simulink library "NMHA_lib"  (Simulink 7.5)
settings: Solver=ode45  StartTime=0.0  StopTime=10.0  RelTol=1e-3
values from neighbouring files (symbols this model uses):
  pNMHA_cnt_CANSleepDely_C = Simulink.Parameter    [NMHA_par.m]
  pNMHA_cnt_VCUSleepDely_C = Simulink.Parameter    [NMHA_par.m]
undefined symbols (not defined in the file or in its folder): p_bool_False_M, p_bool_True_M, VMMCoorrStsTyp
libraries: BaseOperationLib_Browser x6, simulink x1
settings Model: Creator=wuaibin  LastModifiedBy=wuaibin

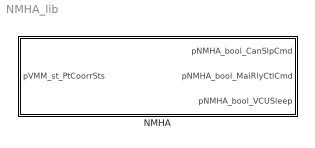
== system NMHA_lib ==
  NMHA : Subsystem  TreatAsAtomicUnit=on

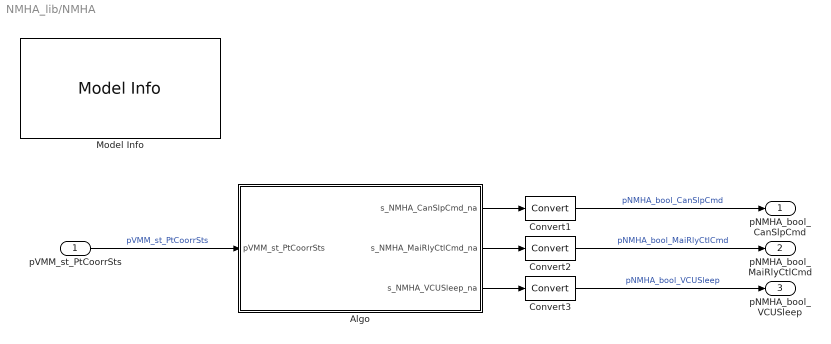
== system NMHA_lib/NMHA ==
  pVMM_st_PtCoorrSts : Inport  OutDataType=fixdt(1, 16)  OutScaling=2^0
  Algo : Subsystem
  Convert1 : DataTypeConversion  OutDataType=fixdt(1, 16)  OutScaling=2^0
  Convert2 : DataTypeConversion  OutDataType=fixdt(1, 16)  OutScaling=2^0
  Convert3 : DataTypeConversion  OutDataType=fixdt(1, 16)  OutScaling=2^0
  Model Info : simulink/Model-Wide Utilities/Model Info  SystemSampleTime=-1  InitialBlockCM=None  BlockCM=None  Frame=on  DisplayStringWithTags=Model Info\nCreated: %<Created>\nCreator: wuaibin  HorizontalTextAlignment=Center  LeftAlignmentValue=0.5  SourceBlockDiagram=HQEV_HCU  TagMaxNumber=20
  pNMHA_bool_CanSlpCmd : Outport  OutDataType=fixdt(1, 16)  OutScaling=2^0
  pNMHA_bool_MaiRlyCtlCmd : Outport  Port=2  OutDataType=fixdt(1, 16)  OutScaling=2^0
  pNMHA_bool_VCUSleep : Outport  Port=3  OutDataType=fixdt(1, 16)  OutScaling=2^0
  wires:
  pVMM_st_PtCoorrSts/1 -> Algo/1(pVMM_st_PtCoorrSts)  "pVMM_st_PtCoorrSts"
  Algo/1(s_NMHA_CanSlpCmd_na) -> Convert1/1
  Convert1/1 -> pNMHA_bool_CanSlpCmd/1  "pNMHA_bool_CanSlpCmd"
  Algo/2(s_NMHA_MaiRlyCtlCmd_na) -> Convert2/1
  Convert2/1 -> pNMHA_bool_MaiRlyCtlCmd/1  "pNMHA_bool_MaiRlyCtlCmd"
  Algo/3(s_NMHA_VCUSleep_na) -> Convert3/1
  Convert3/1 -> pNMHA_bool_VCUSleep/1  "pNMHA_bool_VCUSleep"

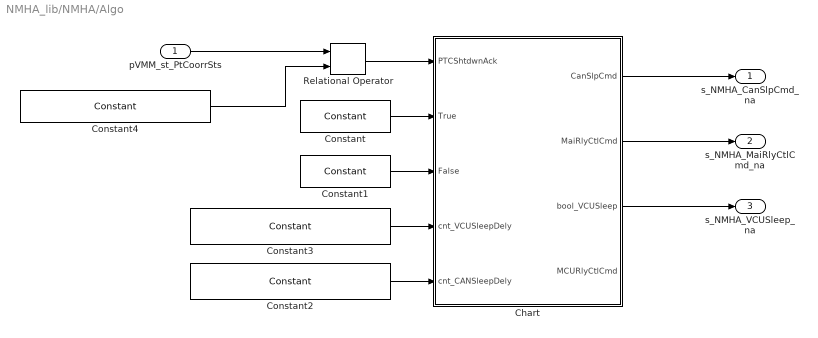
== system NMHA_lib/NMHA/Algo ==
  pVMM_st_PtCoorrSts : Inport  OutDataType=fixdt(1, 16)  OutScaling=2^0
  Chart : Stateflow chart  TreatAsAtomicUnit=on
  Constant : BaseOperationLib_Browser/Sources&Sinks/Constant  Value=p_bool_True_M  OutMin=[]  OutMax=[]  OutDataType=fixdt(1, 16)  ConRadixGroup=Use specified scaling  OutScaling=2^0  OutDataTypeStr=Inherit: Inherit from 'Constant value'
  Constant1 : BaseOperationLib_Browser/Sources&Sinks/Constant  Value=p_bool_False_M  OutMin=[]  OutMax=[]  OutDataType=fixdt(1, 16)  ConRadixGroup=Use specified scaling  OutScaling=2^0  OutDataTypeStr=Inherit: Inherit from 'Constant value'
  Constant2 : BaseOperationLib_Browser/Sources&Sinks/Constant  Value=pNMHA_cnt_CANSleepDely_C  OutMin=[]  OutMax=[]  OutDataType=fixdt(1, 16)  ConRadixGroup=Use specified scaling  OutScaling=2^0  OutDataTypeStr=Inherit: Inherit from 'Constant value'
  Constant3 : BaseOperationLib_Browser/Sources&Sinks/Constant  Value=pNMHA_cnt_VCUSleepDely_C  OutMin=[]  OutMax=[]  OutDataType=fixdt(1, 16)  ConRadixGroup=Use specified scaling  OutScaling=2^0  OutDataTypeStr=Inherit: Inherit from 'Constant value'
  Constant4 : BaseOperationLib_Browser/Sources&Sinks/Constant  Value=uint8(VMMCoorrStsTyp.VMM_LvPwrOff)  OutMin=[]  OutMax=[]  OutDataType=fixdt(1, 16)  ConRadixGroup=Use specified scaling  OutScaling=2^0  OutDataTypeStr=Inherit: Inherit from 'Constant value'
  Relational Operator : BaseOperationLib_Browser/Logic Operations Changed/Relational Operator  Operator===  InputSameDT=on  LogicOutDataTypeMode=Specify via dialog  LogicDataType=PDT_Bool  OutDataTypeStr=PDT_Bool
  s_NMHA_CanSlpCmd_na : Outport  OutDataType=fixdt(1, 16)  OutScaling=2^0
  s_NMHA_MaiRlyCtlCmd_na : Outport  Port=2  OutDataType=fixdt(1, 16)  OutScaling=2^0
  s_NMHA_VCUSleep_na : Outport  Port=3  OutDataType=fixdt(1, 16)  OutScaling=2^0
  wires:
  Constant4/1 -> Relational Operator/2
  Relational Operator/1 -> Chart/1(PTCShtdwnAck)
  pVMM_st_PtCoorrSts/1 -> Relational Operator/1
  Chart/1(CanSlpCmd) -> s_NMHA_CanSlpCmd_na/1
  Chart/2(MaiRlyCtlCmd) -> s_NMHA_MaiRlyCtlCmd_na/1
  Chart/3(bool_VCUSleep) -> s_NMHA_VCUSleep_na/1
  Constant/1 -> Chart/2(True)
  Constant1/1 -> Chart/3(False)
  Constant2/1 -> Chart/5(cnt_CANSleepDely)
  Constant3/1 -> Chart/4(cnt_VCUSleepDely)

== stateflow chart NMHA/Algo/Chart ==
  state VCUSleep
    en:
    cnt=0;
    MaiRlyCtlCmd=False;
    bool_VCUSleep=True;
  state MainRelyOpen
    en:
    cnt=0;
    MaiRlyCtlCmd=False;
    MCURlyCtlCmd=false;
    CanSlpCmd=True;
    bool_VCUSleep=False;
    du:
    cnt++;
  state CANSleep
    en:
    MCURlyCtlCmd=false;
    CanSlpCmd=True;
    du:
    cnt++;
  state Default
    en:
    cnt=0;
    MaiRlyCtlCmd=True;
    CanSlpCmd=False;
    bool_VCUSleep=False;
    MCURlyCtlCmd=true;
  (default) -> MainRelyOpen
  MainRelyOpen -> VCUSleep [order 1] : [cnt>=cnt_VCUSleepDely]
  MainRelyOpen -> Default [order 2] : [PTCShtdwnAck==False]
  CANSleep -> Default [order 2] : [PTCShtdwnAck==False]
  Default -> CANSleep : [PTCShtdwnAck==True]
  CANSleep -> MainRelyOpen [order 1] : [cnt>=cnt_CANSleepDely]
  data: PTCShtdwnAck input double; CanSlpCmd output boolean; MaiRlyCtlCmd output boolean; bool_VCUSleep output boolean; cnt local double; True input double; False input double; cnt_VCUSleepDely input double; cnt_CANSleepDely input double; MCURlyCtlCmd output boolean
